simulink library "ACCI_lib"  (Simulink 7.5)
settings: Solver=ode45  StartTime=0.0  StopTime=10.0  RelTol=1e-3
values from neighbouring files (symbols this model uses):
  pACCI_mV_CCBtnVolt_TAB = Simulink.Parameter    [ACCI_par.m]
  pACCI_Nm_ACCDefaltTrq_C = Simulink.Parameter    [ACCI_par.m]
  pACCI_Nm_ACCMaxTrqReq_C = Simulink.Parameter    [ACCI_par.m]
  pACCI_pct_AEBFact100_C = Simulink.Parameter    [ACCI_par.m]
  pACCI_ratio_AEBFactRateLo_C = Simulink.Parameter    [ACCI_par.m]
  pACCI_ratio_AEBFactRateUp_C = Simulink.Parameter    [ACCI_par.m]
  pACCI_s_ACCBtnIdfyTi_C = Simulink.Parameter    [ACCI_par.m]
  pACCI_st_CCBtnSt_CUR = Simulink.Parameter    [ACCI_par.m]
undefined symbols (not defined in the file or in its folder): ACCStDecelReq, ACCStTrqReq, ACCStTyp, DiscIntNeverNeededParam, p_bool_False_M, p_bool_True_M
libraries: BaseOperationLib_Browser x35, PES_CZ_FAW x2
settings Model: Creator=wuaibin  LastModifiedBy=wuaibin

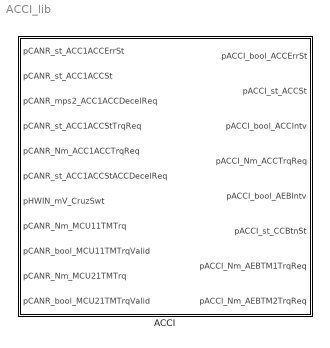
== system ACCI_lib ==
  ACCI : Subsystem

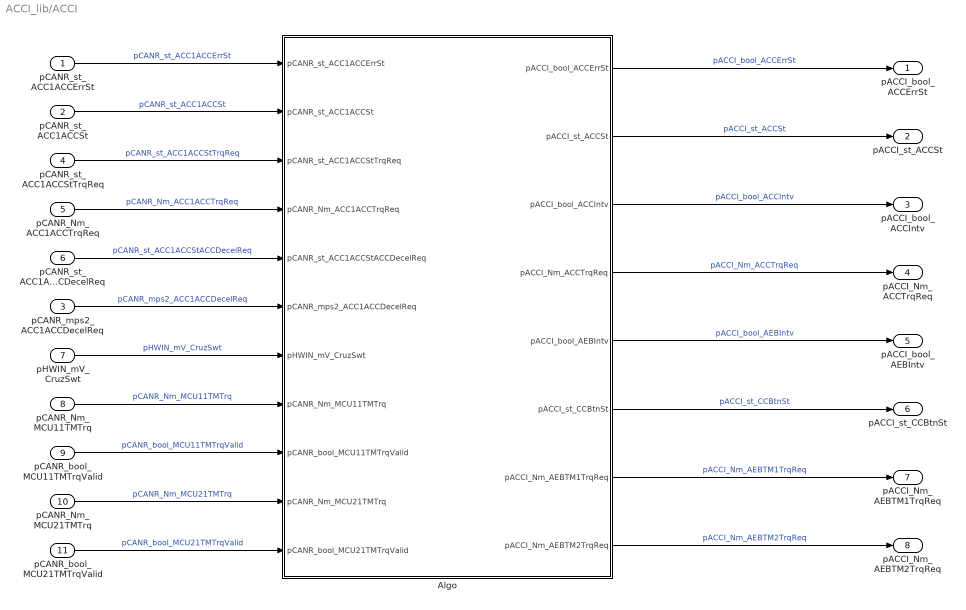
== system ACCI_lib/ACCI ==
  pCANR_st_ACC1ACCErrSt : Inport
  pCANR_st_ACC1ACCSt : Inport  Port=2
  pCANR_mps2_ACC1ACCDecelReq : Inport  Port=3
  pCANR_st_ACC1ACCStTrqReq : Inport  Port=4
  pCANR_Nm_ACC1ACCTrqReq : Inport  Port=5
  pCANR_st_ACC1ACCStACCDecelReq : Inport  Port=6
  pHWIN_mV_CruzSwt : Inport  Port=7
  pCANR_Nm_MCU11TMTrq : Inport  Port=8
  pCANR_bool_MCU11TMTrqValid : Inport  Port=9
  pCANR_Nm_MCU21TMTrq : Inport  Port=10
  pCANR_bool_MCU21TMTrqValid : Inport  Port=11
  Algo : Subsystem
  pACCI_bool_ACCErrSt : Outport  OutDataType=fixdt(1, 16)  OutScaling=2^0
  pACCI_st_ACCSt : Outport  Port=2  OutDataType=fixdt(1, 16)  OutScaling=2^0
  pACCI_bool_ACCIntv : Outport  Port=3  OutDataType=fixdt(1, 16)  OutScaling=2^0
  pACCI_Nm_ACCTrqReq : Outport  Port=4  OutDataType=fixdt(1, 16)  OutScaling=2^0
  pACCI_bool_AEBIntv : Outport  Port=5  OutDataType=fixdt(1, 16)  OutScaling=2^0
  pACCI_st_CCBtnSt : Outport  Port=6  OutDataType=fixdt(1, 16)  OutScaling=2^0
  pACCI_Nm_AEBTM1TrqReq : Outport  Port=7  OutDataType=fixdt(1, 16)  OutScaling=2^0
  pACCI_Nm_AEBTM2TrqReq : Outport  Port=8  OutDataType=fixdt(1, 16)  OutScaling=2^0
  wires:
  Algo/8(pACCI_Nm_AEBTM2TrqReq) -> pACCI_Nm_AEBTM2TrqReq/1  "pACCI_Nm_AEBTM2TrqReq"
  Algo/7(pACCI_Nm_AEBTM1TrqReq) -> pACCI_Nm_AEBTM1TrqReq/1  "pACCI_Nm_AEBTM1TrqReq"
  pCANR_bool_MCU21TMTrqValid/1 -> Algo/11(pCANR_bool_MCU21TMTrqValid)  "pCANR_bool_MCU21TMTrqValid"
  pCANR_Nm_MCU21TMTrq/1 -> Algo/10(pCANR_Nm_MCU21TMTrq)  "pCANR_Nm_MCU21TMTrq"
  pCANR_bool_MCU11TMTrqValid/1 -> Algo/9(pCANR_bool_MCU11TMTrqValid)  "pCANR_bool_MCU11TMTrqValid"
  pCANR_Nm_MCU11TMTrq/1 -> Algo/8(pCANR_Nm_MCU11TMTrq)  "pCANR_Nm_MCU11TMTrq"
  pHWIN_mV_CruzSwt/1 -> Algo/7(pHWIN_mV_CruzSwt)  "pHWIN_mV_CruzSwt"
  Algo/6(pACCI_st_CCBtnSt) -> pACCI_st_CCBtnSt/1  "pACCI_st_CCBtnSt"
  pCANR_mps2_ACC1ACCDecelReq/1 -> Algo/6(pCANR_mps2_ACC1ACCDecelReq)  "pCANR_mps2_ACC1ACCDecelReq"
  Algo/5(pACCI_bool_AEBIntv) -> pACCI_bool_AEBIntv/1  "pACCI_bool_AEBIntv"
  pCANR_st_ACC1ACCStACCDecelReq/1 -> Algo/5(pCANR_st_ACC1ACCStACCDecelReq)  "pCANR_st_ACC1ACCStACCDecelReq"
  Algo/4(pACCI_Nm_ACCTrqReq) -> pACCI_Nm_ACCTrqReq/1  "pACCI_Nm_ACCTrqReq"
  pCANR_Nm_ACC1ACCTrqReq/1 -> Algo/4(pCANR_Nm_ACC1ACCTrqReq)  "pCANR_Nm_ACC1ACCTrqReq"
  pCANR_st_ACC1ACCStTrqReq/1 -> Algo/3(pCANR_st_ACC1ACCStTrqReq)  "pCANR_st_ACC1ACCStTrqReq"
  Algo/3(pACCI_bool_ACCIntv) -> pACCI_bool_ACCIntv/1  "pACCI_bool_ACCIntv"
  pCANR_st_ACC1ACCSt/1 -> Algo/2(pCANR_st_ACC1ACCSt)  "pCANR_st_ACC1ACCSt"
  Algo/2(pACCI_st_ACCSt) -> pACCI_st_ACCSt/1  "pACCI_st_ACCSt"
  Algo/1(pACCI_bool_ACCErrSt) -> pACCI_bool_ACCErrSt/1  "pACCI_bool_ACCErrSt"
  pCANR_st_ACC1ACCErrSt/1 -> Algo/1(pCANR_st_ACC1ACCErrSt)  "pCANR_st_ACC1ACCErrSt"

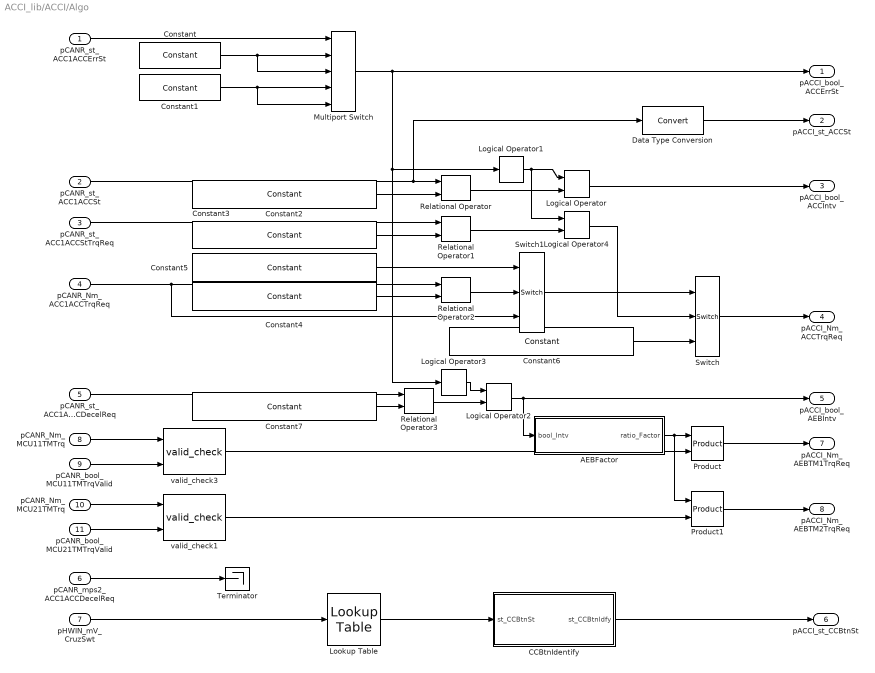
== system ACCI_lib/ACCI/Algo ==
  pCANR_st_ACC1ACCErrSt : Inport
  pCANR_st_ACC1ACCSt : Inport  Port=2
  pCANR_st_ACC1ACCStTrqReq : Inport  Port=3
  pCANR_Nm_ACC1ACCTrqReq : Inport  Port=4
  pCANR_st_ACC1ACCStACCDecelReq : Inport  Port=5
  pCANR_mps2_ACC1ACCDecelReq : Inport  Port=6
  pHWIN_mV_CruzSwt : Inport  Port=7
  pCANR_Nm_MCU11TMTrq : Inport  Port=8
  pCANR_bool_MCU11TMTrqValid : Inport  Port=9
  pCANR_Nm_MCU21TMTrq : Inport  Port=10
  pCANR_bool_MCU21TMTrqValid : Inport  Port=11
  AEBFactor : Subsystem
  CCBtnIdentify : Subsystem
  Constant : BaseOperationLib_Browser/Sources&Sinks/Constant  Value=p_bool_False_M  OutMin=[]  OutMax=[]  OutDataType=fixdt(1, 16)  ConRadixGroup=Use specified scaling  OutScaling=2^0  OutDataTypeStr=Inherit: Inherit from 'Constant value'
  Constant1 : BaseOperationLib_Browser/Sources&Sinks/Constant  Value=p_bool_True_M  OutMin=[]  OutMax=[]  OutDataType=fixdt(1, 16)  ConRadixGroup=Use specified scaling  OutScaling=2^0  OutDataTypeStr=Inherit: Inherit from 'Constant value'
  Constant2 : BaseOperationLib_Browser/Sources&Sinks/Constant  Value=uint8(ACCStTyp.ACCST_Active)  OutMin=[]  OutMax=[]  OutDataType=Enum: ACCStTyp  ConRadixGroup=Best Precision: Vector-wise  OutScaling=[]  OutDataTypeStr=Inherit: Inherit from 'Constant value'
  Constant3 : BaseOperationLib_Browser/Sources&Sinks/Constant  Value=uint8(ACCStTrqReq.ACCSTR_Req)  OutMin=[]  OutMax=[]  OutDataType=Enum: ACCStTyp  ConRadixGroup=Best Precision: Vector-wise  OutScaling=[]  OutDataTypeStr=Inherit: Inherit from 'Constant value'
  Constant4 : BaseOperationLib_Browser/Sources&Sinks/Constant  Value=pACCI_Nm_ACCMaxTrqReq_C  OutMin=[]  OutMax=[]  OutDataType=Enum: ACCStTyp  ConRadixGroup=Best Precision: Vector-wise  OutScaling=[]  OutDataTypeStr=Inherit: Inherit from 'Constant value'
  Constant5 : BaseOperationLib_Browser/Sources&Sinks/Constant  Value=pACCI_Nm_ACCDefaltTrq_C  OutMin=[]  OutMax=[]  OutDataType=Enum: ACCStTyp  ConRadixGroup=Best Precision: Vector-wise  OutScaling=[]  OutDataTypeStr=Inherit: Inherit from 'Constant value'
  Constant6 : BaseOperationLib_Browser/Sources&Sinks/Constant  Value=pACCI_Nm_ACCDefaltTrq_C  OutMin=[]  OutMax=[]  OutDataType=Enum: ACCStTyp  ConRadixGroup=Best Precision: Vector-wise  OutScaling=[]  OutDataTypeStr=Inherit: Inherit from 'Constant value'
  Constant7 : BaseOperationLib_Browser/Sources&Sinks/Constant  Value=uint8(ACCStDecelReq.ACCSDR_PCS)  OutMin=[]  OutMax=[]  OutDataType=Enum: ACCStTyp  ConRadixGroup=Best Precision: Vector-wise  OutScaling=[]  OutDataTypeStr=Inherit: Inherit from 'Constant value'
  Data Type Conversion : DataTypeConversion  OutDataType=fixdt(1, 16)  OutScaling=2^0
  Logical Operator : BaseOperationLib_Browser/Logic Operations Changed/Logical Operator  Operator=AND  Inputs=2  AllPortsSameDT=on  OutDataTypeMode=Specify via dialog  LogicDataType=PDT_Bool  OutDataTypeStr=PDT_Bool
  Logical Operator1 : BaseOperationLib_Browser/Logic Operations Changed/Logical Operator  Operator=NOT  Inputs=2  AllPortsSameDT=on  OutDataTypeMode=Specify via dialog  LogicDataType=PDT_Bool  OutDataTypeStr=PDT_Bool
  Logical Operator2 : BaseOperationLib_Browser/Logic Operations Changed/Logical Operator  Operator=AND  Inputs=2  AllPortsSameDT=on  OutDataTypeMode=Specify via dialog  LogicDataType=PDT_Bool  OutDataTypeStr=PDT_Bool
  Logical Operator3 : BaseOperationLib_Browser/Logic Operations Changed/Logical Operator  Operator=NOT  Inputs=2  AllPortsSameDT=on  OutDataTypeMode=Specify via dialog  LogicDataType=PDT_Bool  OutDataTypeStr=PDT_Bool
  Logical Operator4 : BaseOperationLib_Browser/Logic Operations Changed/Logical Operator  Operator=AND  Inputs=2  AllPortsSameDT=on  OutDataTypeMode=Specify via dialog  LogicDataType=PDT_Bool  OutDataTypeStr=PDT_Bool
  Lookup Table : BaseOperationLib_Browser/Lookup Tables Changed/Lookup Table  InputValues=pACCI_mV_CCBtnVolt_TAB  Table=pACCI_st_CCBtnSt_CUR  LookUpMeth=Use Input Below  OutMin=[]  OutMax=[]  OutDataType=fixdt(1, 16)  OutScaling=2^0  OutDataTypeStr=Inherit: Inherit via back propagation  SaturateOnIntegerOverflow=on
      settings: AttributesFormatString=X:%<InputValues>\nTAB:%<Table>
  Multiport Switch : BaseOperationLib_Browser/Signal Routing Changed/Multiport Switch  DataPortOrder=Specify indices  Inputs=4  DataPortIndices={uint8(ACC1ErrStTyp.ACCES_NOErr),uint8(ACC1ErrStTyp.ACCES_Derate),uint8(ACC1ErrStTyp.ACCES_Reverse),uint8(ACC1ErrStTyp.ACCES_Err)}  zeroidx=off  InputSameDT=on  OutMin=[]  OutMax=[]  OutDataType=fixdt(1, 16)  OutScaling=2^0  SaturateOnIntegerOverflow=on
  Product : BaseOperationLib_Browser/Math Operations Changed/Product  Inputs=2  Multiplication=Element-wise(.*)  OutMin=[]  OutMax=[]  OutDataType=fixdt(1,16,0)  OutScaling=[]  OutDataTypeStr=Inherit: Inherit via back propagation  RndMeth=Zero  SaturateOnIntegerOverflow=on
  Product1 : BaseOperationLib_Browser/Math Operations Changed/Product  Inputs=2  Multiplication=Element-wise(.*)  OutMin=[]  OutMax=[]  OutDataType=fixdt(1,16,0)  OutScaling=[]  OutDataTypeStr=Inherit: Inherit via back propagation  RndMeth=Zero  SaturateOnIntegerOverflow=on
  Relational Operator : BaseOperationLib_Browser/Logic Operations Changed/Relational Operator  Operator===  InputSameDT=on  LogicOutDataTypeMode=Specify via dialog  LogicDataType=PDT_Bool  OutDataTypeStr=PDT_Bool
  Relational Operator1 : BaseOperationLib_Browser/Logic Operations Changed/Relational Operator  Operator===  InputSameDT=on  LogicOutDataTypeMode=Specify via dialog  LogicDataType=PDT_Bool  OutDataTypeStr=PDT_Bool
  Relational Operator2 : BaseOperationLib_Browser/Logic Operations Changed/Relational Operator  Operator=>=  InputSameDT=on  LogicOutDataTypeMode=Specify via dialog  LogicDataType=PDT_Bool  OutDataTypeStr=PDT_Bool
  Relational Operator3 : BaseOperationLib_Browser/Logic Operations Changed/Relational Operator  Operator===  InputSameDT=on  LogicOutDataTypeMode=Specify via dialog  LogicDataType=PDT_Bool  OutDataTypeStr=PDT_Bool
  Switch : BaseOperationLib_Browser/Signal Routing Changed/Switch  Criteria=u2 ~= 0  Threshold=1  InputSameDT=on  OutMin=[]  OutMax=[]  OutDataType=fixdt(1,16,0)  OutScaling=[]  SaturateOnIntegerOverflow=on
  Switch1 : BaseOperationLib_Browser/Signal Routing Changed/Switch  Criteria=u2 ~= 0  Threshold=1  InputSameDT=on  OutMin=[]  OutMax=[]  OutDataType=fixdt(1,16,0)  OutScaling=[]  SaturateOnIntegerOverflow=on
  Terminator : Terminator
  valid_check1 : PES_CZ_FAW/Discontinuities/valid_check  SystemSampleTime=-1  init=0
  valid_check3 : PES_CZ_FAW/Discontinuities/valid_check  SystemSampleTime=-1  init=0
  pACCI_bool_ACCErrSt : Outport  OutDataType=fixdt(1, 16)  OutScaling=2^0
  pACCI_st_ACCSt : Outport  Port=2  OutDataType=fixdt(1, 16)  OutScaling=2^0
  pACCI_bool_ACCIntv : Outport  Port=3  OutDataType=fixdt(1, 16)  OutScaling=2^0
  pACCI_Nm_ACCTrqReq : Outport  Port=4  OutDataType=fixdt(1, 16)  OutScaling=2^0
  pACCI_bool_AEBIntv : Outport  Port=5  OutDataType=fixdt(1, 16)  OutScaling=2^0
  pACCI_st_CCBtnSt : Outport  Port=6  OutDataType=fixdt(1, 16)  OutScaling=2^0
  pACCI_Nm_AEBTM1TrqReq : Outport  Port=7  OutDataType=fixdt(1, 16)  OutScaling=2^0
  pACCI_Nm_AEBTM2TrqReq : Outport  Port=8  OutDataType=fixdt(1, 16)  OutScaling=2^0
  wires:
  Data Type Conversion/1 -> pACCI_st_ACCSt/1
  valid_check3/1 -> Product/2
  Product1/1 -> pACCI_Nm_AEBTM2TrqReq/1
  valid_check1/1 -> Product1/2
  Product/1 -> pACCI_Nm_AEBTM1TrqReq/1
  AEBFactor/1(ratio_Factor) -> Product1/1, Product/1
  pCANR_bool_MCU21TMTrqValid/1 -> valid_check1/2
  pCANR_Nm_MCU21TMTrq/1 -> valid_check1/1
  pCANR_bool_MCU11TMTrqValid/1 -> valid_check3/2
  pCANR_Nm_MCU11TMTrq/1 -> valid_check3/1
  CCBtnIdentify/1(st_CCBtnIdfy) -> pACCI_st_CCBtnSt/1
  Lookup Table/1 -> CCBtnIdentify/1(st_CCBtnSt)
  pHWIN_mV_CruzSwt/1 -> Lookup Table/1
  pCANR_mps2_ACC1ACCDecelReq/1 -> Terminator/1
  Logical Operator2/1 -> AEBFactor/1(bool_Intv), pACCI_bool_AEBIntv/1
  Logical Operator3/1 -> Logical Operator2/1
  Relational Operator3/1 -> Logical Operator2/2
  pCANR_st_ACC1ACCStACCDecelReq/1 -> Relational Operator3/1
  Constant7/1 -> Relational Operator3/2
  Switch/1 -> pACCI_Nm_ACCTrqReq/1
  Constant6/1 -> Switch/3
  Switch1/1 -> Switch/1
  Constant5/1 -> Switch1/1
  Relational Operator2/1 -> Switch1/2
  Constant4/1 -> Relational Operator2/2
  pCANR_Nm_ACC1ACCTrqReq/1 -> Switch1/3, Relational Operator2/1
  Logical Operator1/1 -> Logical Operator/1, Logical Operator4/1
  Logical Operator/1 -> pACCI_bool_ACCIntv/1
  Relational Operator/1 -> Logical Operator/2
  Constant3/1 -> Relational Operator1/2
  pCANR_st_ACC1ACCStTrqReq/1 -> Relational Operator1/1
  pCANR_st_ACC1ACCSt/1 -> Data Type Conversion/1, Relational Operator/1
  Constant2/1 -> Relational Operator/2
  Constant1/1 -> Multiport Switch/5, Multiport Switch/4
  Constant/1 -> Multiport Switch/3, Multiport Switch/2
  Multiport Switch/1 -> Logical Operator3/1, Logical Operator1/1, pACCI_bool_ACCErrSt/1
  pCANR_st_ACC1ACCErrSt/1 -> Multiport Switch/1
  Relational Operator1/1 -> Logical Operator4/2
  Logical Operator4/1 -> Switch/2

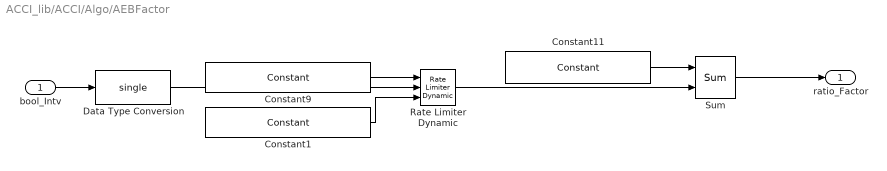
== system ACCI_lib/ACCI/Algo/AEBFactor ==
  bool_Intv : Inport  OutDataType=fixdt(1, 16)  OutScaling=2^0
  Constant1 : BaseOperationLib_Browser/Sources&Sinks/Constant  Value=pACCI_ratio_AEBFactRateLo_C  OutMin=[]  OutMax=[]  OutDataType=fixdt(1, 16)  ConRadixGroup=Use specified scaling  OutScaling=2^0  OutDataTypeStr=Inherit: Inherit from 'Constant value'
  Constant11 : BaseOperationLib_Browser/Sources&Sinks/Constant  Value=pACCI_pct_AEBFact100_C  OutMin=[]  OutMax=[]  OutDataType=fixdt(1, 16)  ConRadixGroup=Use specified scaling  OutScaling=2^0  OutDataTypeStr=Inherit: Inherit from 'Constant value'
  Constant9 : BaseOperationLib_Browser/Sources&Sinks/Constant  Value=pACCI_ratio_AEBFactRateUp_C  OutMin=[]  OutMax=[]  OutDataType=fixdt(1, 16)  ConRadixGroup=Use specified scaling  OutScaling=2^0  OutDataTypeStr=Inherit: Inherit from 'Constant value'
  Data Type Conversion : DataTypeConversion  OutDataTypeMode=single  OutDataType=fixdt(1, 16)  OutScaling=2^0  OutDataTypeStr=single
  Rate Limiter Dynamic : BaseOperationLib_Browser/Discontinuities Unchanged/Rate Limiter Dynamic  SystemSampleTime=-1
  Sum : BaseOperationLib_Browser/Math Operations Changed/Sum  Inputs=+-  InputSameDT=on  OutMin=[]  OutMax=[]  OutDataType=fixdt(1, 16)  OutScaling=2^0  SaturateOnIntegerOverflow=on
  ratio_Factor : Outport  OutDataType=fixdt(1, 16)  OutScaling=2^0
  wires:
  bool_Intv/1 -> Data Type Conversion/1
  Sum/1 -> ratio_Factor/1
  Data Type Conversion/1 -> Rate Limiter Dynamic/2
  Constant9/1 -> Rate Limiter Dynamic/1
  Constant1/1 -> Rate Limiter Dynamic/3
  Rate Limiter Dynamic/1 -> Sum/2
  Constant11/1 -> Sum/1

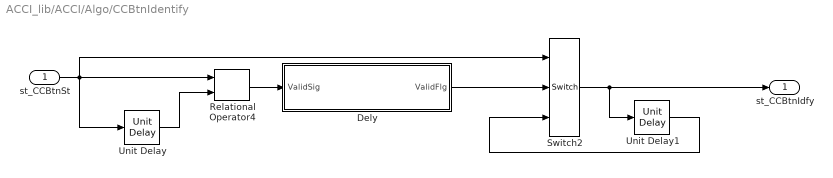
== system ACCI_lib/ACCI/Algo/CCBtnIdentify ==
  st_CCBtnSt : Inport
  Dely : Subsystem  mask{timeoutthres=pACCI_s_ACCBtnIdfyTi_C}
      mask prompts: timeoutthres "Timeout counter Treshold"
      mask help:
      | WatchDog block
      |
      | If input bool signal is false for the number of step bigger than "Timeout counter Threshold" the output WatchDog signal is set to True.
      |
      | Tip. Set the thresshold to the required time in seconds devided by algorithm sampling time.
      mask Help:
      | WatchDog block
      | 
      | If input bool signal is false for the number of step bigger than "Timeout counter Threshold" the output WatchDog signal is set to True.
      | 
      | Tip. Set the thresshold to required time in second devided by sampling time.
  Relational Operator4 : BaseOperationLib_Browser/Logic Operations Changed/Relational Operator  Operator===  InputSameDT=on  LogicOutDataTypeMode=Specify via dialog  LogicDataType=PDT_Bool  OutDataTypeStr=PDT_Bool
  Switch2 : BaseOperationLib_Browser/Signal Routing Changed/Switch  Criteria=u2 ~= 0  Threshold=1  InputSameDT=on  OutMin=[]  OutMax=[]  OutDataType=fixdt(1,16,0)  OutScaling=[]  SaturateOnIntegerOverflow=on
  Unit Delay : BaseOperationLib_Browser/Discrete Unchanged /Unit Delay  X0=0  SampleTime=-1
  Unit Delay1 : BaseOperationLib_Browser/Discrete Unchanged /Unit Delay  X0=0  SampleTime=-1
  st_CCBtnIdfy : Outport
  wires:
  Unit Delay1/1 -> Switch2/3
  Switch2/1 -> st_CCBtnIdfy/1, Unit Delay1/1
  Dely/1(ValidFlg) -> Switch2/2
  Unit Delay/1 -> Relational Operator4/2
  Relational Operator4/1 -> Dely/1(ValidSig)
  st_CCBtnSt/1 -> Unit Delay/1, Relational Operator4/1, Switch2/1

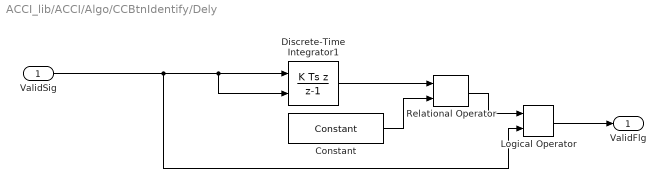
== system ACCI_lib/ACCI/Algo/CCBtnIdentify/Dely ==
  ValidSig : Inport  OutDataType=fixdt(1, 16)  OutScaling=2^0
  Constant : BaseOperationLib_Browser/Sources&Sinks/Constant  Value=timeoutthres  OutMin=[]  OutMax=[]  OutDataType=fixdt(1, 16)  ConRadixGroup=Use specified scaling  OutScaling=2^0  OutDataTypeStr=Inherit: Inherit from 'Constant value'
  Discrete-Time Integrator1 : DiscreteIntegrator  IntegratorMethod=Integration: Backward Euler  ExternalReset=rising  SampleTime=-1  OutDataType=PDT_s  OutDataTypeStr=Inherit: Inherit via back propagation  UpperSaturationLimit=100  LowerSaturationLimit=0  ICPrevOutput=DiscIntNeverNeededParam  ICPrevScaledInput=DiscIntNeverNeededParam
  Logical Operator : BaseOperationLib_Browser/Logic Operations Changed/Logical Operator  Operator=AND  Inputs=2  AllPortsSameDT=on  OutDataTypeMode=Specify via dialog  LogicDataType=PDT_Bool  OutDataTypeStr=PDT_Bool
  Relational Operator : BaseOperationLib_Browser/Logic Operations Changed/Relational Operator  Operator=>=  InputSameDT=on  LogicOutDataTypeMode=Specify via dialog  LogicDataType=PDT_Bool  OutDataTypeStr=PDT_Bool
  ValidFlg : Outport  OutDataType=fixdt(1, 16)  OutScaling=2^0
  wires:
  Discrete-Time Integrator1/1 -> Relational Operator/1
  Constant/1 -> Relational Operator/2
  Logical Operator/1 -> ValidFlg/1
  Relational Operator/1 -> Logical Operator/1
  ValidSig/1 -> Logical Operator/2, Discrete-Time Integrator1/2, Discrete-Time Integrator1/1
